simulink model "lab322"  (R2022a)
settings: Solver=VariableStepAuto  StartTime=0.0  StopTime=1  MaxStep=1e-3  RelTol=1e-3
undefined symbols (not defined in the file): ACsource, Angle, D1, lagging, Phase, pulse, RaLa, RbLb, RcLc, RL
libraries: spsThyristorLib x6, spsFourierLib x5, spsVoltageMeasurementLib x5, spsSeriesRLCBranchLib x4, spsACVoltageSourceLib x3, spsCurrentMeasurementLib x2, spsGroundLib x1, spsRMSLib x1, simulink x1, spsPLL3phLib x1, spsPulseGeneratorThyristor12PulseLib x1, spsThreePhaseVIMeasurementLib x1
settings Model: Creator=Viktor  LastModifiedBy=админ
settings ModelReferenceCC: EnableRefExpFcnMdlSchedulingChecks=off
settings RTWCC: Description=Generic Real-Time Target  GPUComputeCapability=5.0

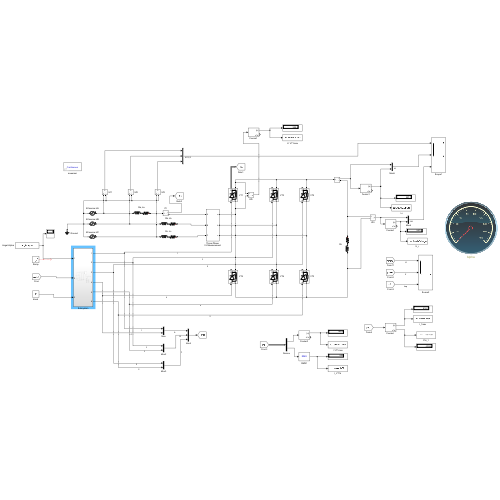
[thumbnail: Simulink's stored preview of the top-level diagram]
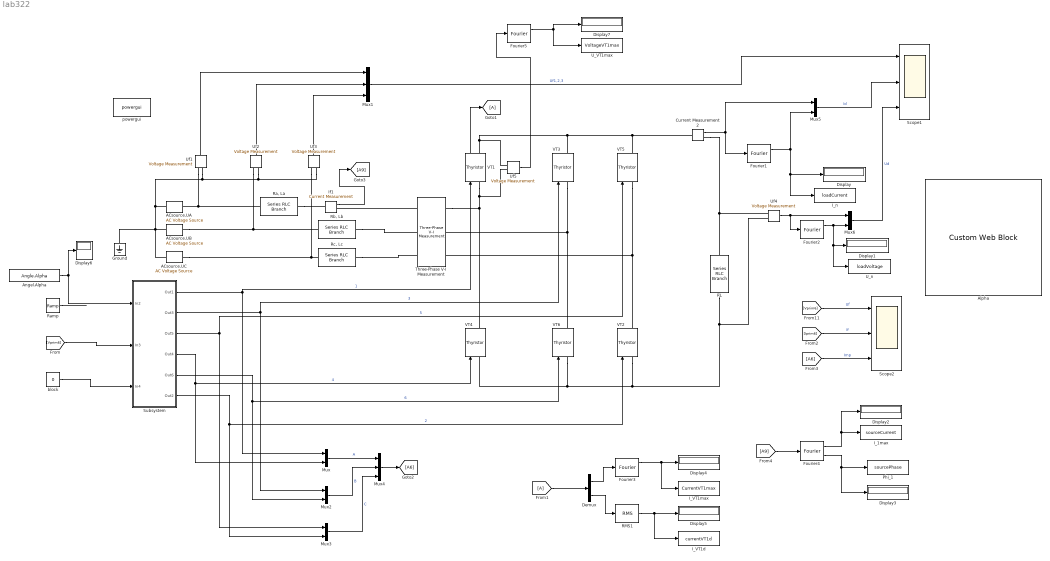
== system lab322 ==
  ACsource.UA : spsACVoltageSourceLib/AC Voltage Source  Amplitude=ACsource.U_A  Phase=Phase.A  Frequency=ACsource.f_c  SampleTime=0  Measurements=None  BusType=swing  Pref=10e3  Qref=0  Qmin=-inf  Qmax=+inf
  ACsource.UB : spsACVoltageSourceLib/AC Voltage Source  Amplitude=ACsource.U_B  Phase=Phase.B  Frequency=ACsource.f_c  SampleTime=0  Measurements=None  BusType=swing  Pref=10e3  Qref=0  Qmin=-inf  Qmax=+inf
  ACsource.UC : spsACVoltageSourceLib/AC Voltage Source  Amplitude=ACsource.U_C  Phase=Phase.C  Frequency=ACsource.f_c  SampleTime=0  Measurements=None  BusType=swing  Pref=10e3  Qref=0  Qmin=-inf  Qmax=+inf
  Alpha : CustomWebBlock  LabelPosition=Hide  ShowInitialText=on  Configuration="{\"components\":[{\"name\":\"CircularScaleComponent\",\"settings\":{\"bounds\":{\"max\":180,\"min\":0,\"tickInterval\":\"auto\"},\"direction\":\"cw\",\"flipLimits\":0,\"innerRadius\":0.75,\"internalTickHeightScaleFactor\":1,\"labelColor\":[255,255,200],\"labelFont\":{\"font\":\"Arial\",\"fontSize\":12},\"labelTransparency\":1,\"minorTickHeightScaleFactor\":0.2,\"needleImage\":{\"size\":[200,50],\"src\":\"data:image\\/svg+xml;base64,PD94bWwgdmVyc2lvbj0iMS4wIiBlbmNvZGluZz0idXRmLTgiPz4KPCEtLSBHZW5lcmF0b3I6IEFkb2JlIElsbHVzdHJhdG9yIDI0LjEuMiwgU1ZHIEV4cG9ydCBQbHVnLUluIC4gU1ZHIFZlcnNpb246IDYuMDAgQnVpbGQgMCkgIC0tPgo8c3ZnIHZlcnNpb249IjEuMSIgaWQ9IkxheWVyXzEiIHhtbG5zPSJodHRwOi8vd3d3LnczLm9yZy8yMDAwL3N2ZyIgeG1sbnM6eGxpbms9Imh0dHA6Ly93d3cudzMub3JnLzE5OTkveGxpbmsiIHg9IjBweCIgeT0iMHB4IgoJIHZpZXdCb3g9IjAgMCAyMDAgNTAiIHN0eWxlPSJlbmFibGUtYmFja2dyb3VuZDpuZXcgMCAwIDIwMCA1MDsiIHhtbDpzcGFjZT0icHJlc2VydmUiPgo8c3R5bGUgdHlwZT0idGV4dC9jc3MiPgoJLnN0MHtmaWxsOiNFQzIxMjc7fQo8L3N0eWxlPgo8cGF0aCBjbGFzcz0ic3QwIiBkPSJNMTYyLjgsMTMuN0MxNjksNC40LDE4MS43LDEuOSwxOTEsOC4xczExLjgsMTguOSw1LjYsMjguMnMtMTguOSwxMS44LTI4LjIsNS42bDAsMAoJQzE1OS4xLDM1LjYsMTU2LjYsMjMsMTYyLjgsMTMuN0wxNjIuOCwxMy43eiBNMTY1LjgsMTUuOGMtNS4xLDcuNi0zLjEsMTcuOSw0LjYsMjNjNy42LDUuMSwxNy45LDMuMSwyMy00LjYKCWM1LjEtNy42LDMuMS0xNy45LTQuNi0yM2wwLDBDMTgxLjIsNi4yLDE3MC45LDguMiwxNjUuOCwxNS44eiIvPgo8cGF0aCBjbGFzcz0ic3QwIiBkPSJNMC40LDI1Ljl2LTMuM2wxNTktMi41Yy0wLjcsMi42LTAuNyw1LjIsMCw3LjhMMC40LDI1Ljl6Ii8+CjxjaXJjbGUgY2xhc3M9InN0MCIgY3g9IjE3OS42IiBjeT0iMjQiIHI9IjAuNyIvPgo8L3N2Zz4K\"},\"needleOffset\":[0.18464878250906522,0],\"needleOrientation\":-45,\"needleRotation\":180,\"needleSize\":{\"height\":0.11741692305346914,\"width\":0.46108337545091255},\"outerRadius\":0.9,\"position\":[0.06486742424242424,0.05627705627705628,0.8917748917748918,0.8787878787878788],\"referencePoint\":\"auto\",\"scaleAngle\":270,\"scaleAngleOffset\":135,\"scaleColors\":[{\"color\":[162,20,47],\"max\":0,\"min\":0}],\"scaleColorsSize\":0.2,\"scaleDirection\":\"CW\",\"scalePosition\":[0,0,1,1],\"showLabels\":1,\"showMinorTicks\":1,\"showSpanLine\":1,\"showTicks\":1,\"tickColor\":[252,252,197],\"tickTransparency\":1,\"valueBarColor\":[217,83,25],\"valueBarPosition\":[0,0,1,1],\"valueBarSize\":0.2,\"valueBarTransparency\":1}},{\"name\":\"BackgroundImageComponent\",\"settings\":{\"image\":{\"size\":[500,500],\"src\":\"data:image\\/svg+xml;base64,PD94bWwgdmVyc2lvbj0iMS4wIiBlbmNvZGluZz0iVVRGLTgiIHN0YW5kYWxvbmU9Im5vIj8+CjxzdmcKICAgeG1sbnM6ZGM9Imh0dHA6Ly9wdXJsLm9yZy9kYy9lbGVtZW50cy8xLjEvIgogICB4bWxuczpjYz0iaHR0cDovL2NyZWF0aXZlY29tbW9ucy5vcmcvbnMjIgogICB4bWxuczpyZGY9Imh0dHA6Ly93d3cudzMub3JnLzE5OTkvMDIvMjItcmRmLXN5bnRheC1ucyMiCiAgIHhtbG5zOnN2Zz0iaHR0cDovL3d3dy53My5vcmcvMjAwMC9zdmciCiAgIHhtbG5zPSJodHRwOi8vd3d3LnczLm9yZy8yMDAwL3N2ZyIKICAgeG1sbnM6 ...(+9964 chars)\"},\"position\":[0,0,1,1],\"scaleMode\":\"0\"}},{\"name\":\"ForegroundImageComponent\",\"settings\":{\"image\":{\"size\":[0,0],\"src\":\"default\",\"srcOrientation\":[]},\"isForeground\":1,\"position\":[0,0,1,1],\"scaleMode\":\"0\"}}],\"settings\":{\"BindingType\":\"signal\",\"aspectRatio\":1.032258064516129,\"backgroundColor\":[0,0,0,\"1\"],\"backgroundOffset\":0.14,\"backgroundOpacity\":1,\"direction\":\"cw\",\"fixedAspectRatio\":\"on\",\"flipLimits\":0,\"orientation\":\"horizontal\",\"showBackgroundColor\":false,\"value\":0},\"type\":\"CircularGauge\"}"
  Angel.Alpha : Constant  Value=Angle.Alpha
  Current Measurement2 : spsCurrentMeasurementLib/Current Measurement  PhasorSimulation=off  OutputType=Complex  PSBequivalent=0
  Demux : Demux  Outputs=2
  Display{,1..7} (8 alike) : Display
  Fourier1 : spsFourierLib/Fourier  Freq=ACsource.f_c  n=0  InInit=[0, 0]  Ts=0
      settings: SourceProductBaseCode=PS
  Fourier2 : spsFourierLib/Fourier  Freq=ACsource.f_c  n=0  InInit=[0, 0]  Ts=0
      settings: SourceProductBaseCode=PS
  Fourier3 : spsFourierLib/Fourier  Freq=ACsource.f_c  n=0  InInit=[0, 0]  Ts=0
      settings: SourceProductBaseCode=PS
  Fourier4 : spsFourierLib/Fourier  Freq=ACsource.f_c  n=1  InInit=[0, 0]  Ts=0
      settings: SourceProductBaseCode=PS
  Fourier5 : spsFourierLib/Fourier  Freq=ACsource.f_c  n=1  InInit=[0, 0]  Ts=0
      settings: SourceProductBaseCode=PS
  From1 : From
  Goto1 : Goto
  Ground : spsGroundLib/Ground  LConnTagsString=a
  I_1max : ToWorkspace  VariableName=sourceCurrent  SampleTime=-1
  I_VT1d : ToWorkspace  VariableName=currentVT1d  SampleTime=-1
  I_VT1max : ToWorkspace  VariableName=CurrentVT1max  SampleTime=-1
  I_n : ToWorkspace  VariableName=loadCurrent  SampleTime=-1
  If1 : spsCurrentMeasurementLib/Current Measurement  PhasorSimulation=off  OutputType=Complex  PSBequivalent=0
  Mux{,2..3,5..6} (5 alike) : Mux  Inputs=2
  Mux1 : Mux  Inputs=3
  Mux4 : Mux  Inputs=3
  Phi_1 : ToWorkspace  VariableName=sourcePhase  SampleTime=-1
      settings: Save2DSignal=2-D array (concatenate along first dimension)
  RL : spsSeriesRLCBranchLib/Series RLC Branch  LConnTagsString=__new0  RConnTagsString=__new0  BranchType=RL  Resistance=RL.Res  Inductance=RL.Ind  SetiL0=off  InitialCurrent=0  Capacitance=1e-6  Setx0=off  InitialVoltage=0  Measurements=None
  RMS1 : spsRMSLib/RMS  TrueRMS=on  Freq=ACsource.U_A  RMSInit=0  Ts=0
  "Ra, La" : spsSeriesRLCBranchLib/Series RLC Branch  LConnTagsString=__new0  RConnTagsString=__new0  BranchType=RL  Resistance=RaLa.Res  Inductance=RaLa.Ind  SetiL0=off  InitialCurrent=0  Capacitance=1e-6  Setx0=off  InitialVoltage=0  Measurements=None
  Ramp : simulink/Sources/Ramp  slope=1  start=0  InitialOutput=0
  "Rb, Lb" : spsSeriesRLCBranchLib/Series RLC Branch  LConnTagsString=__new0  RConnTagsString=__new0  BranchType=RL  Resistance=RbLb.Res  Inductance=RbLb.Ind  SetiL0=off  InitialCurrent=0  Capacitance=1e-6  Setx0=off  InitialVoltage=0  Measurements=None
  "Rc, Lc" : spsSeriesRLCBranchLib/Series RLC Branch  LConnTagsString=__new0  RConnTagsString=__new0  BranchType=RL  Resistance=RcLc.Res  Inductance=RcLc.Ind  SetiL0=off  InitialCurrent=0  Capacitance=1e-6  Setx0=off  InitialVoltage=0  Measurements=None
  Scope1 : Scope  NumInputPorts=3
  Scope2 : Scope  NumInputPorts=3
  Subsystem : Subsystem
  Three-Phase V-I Measurement : spsThreePhaseVIMeasurementLib/Three-Phase V-I Measurement  VoltageMeasurement=phase-to-ground  SetLabelV=on  LabelV=Vprim6  Vpu=off  VpuLL=off  CurrentMeasurement=yes  SetLabelI=on  LabelI=Iprim6  Ipu=off  Pbase=100e6  Vbase=500e3  OutputType=Complex  PhasorSimulation=off  PSBequivalent=0
  U_VT1max : ToWorkspace  VariableName=VoltageVT1max  SampleTime=-1
  U_n : ToWorkspace  VariableName=loadVoltage  SampleTime=0.002
  Uf{1..5} (5 alike) : spsVoltageMeasurementLib/Voltage Measurement  PhasorSimulation=off  OutputType=Complex  PSBequivalent=0
  VT{1..6} (6 alike) : spsThyristorLib/Thyristor  Ron=VT.Res  Lon=0  Vf=VT.U_f  IC=0  Rs=500  Cs=250e-9  Measurements=on
  block : Constant  Value=0
  powergui : spspowerguiLib/powergui  Priority=1  SimulationMode=Continuous  SampleTime=50e-6  frequency=60  Iterations=50  frequencyindice=0  Pbase=100e6  ErrMax=1e-4  UnitsV=kV  UnitsW=MW  buscounter=0  FunctionMessages=off  echomessages=off  EnableUseOfTLC=off  CurrentSourceSwitches=off  DisableSnubberDevices=off  DisableRonSwitches=off  DisableVfSwitches=off  DisplayEquations=off  AutomaticDiscreteSolvers=off  SolverType=Tustin/Backward Euler (TBE)  Interpol=off  ExternalGateDelay=off  methode=off  Ts=100  x0status=blocks  SPID=on  SwTol=0  HookPort=off  NonlinearTolerance=1e-4  nMaxIteration=100  ContinueOnMaxIteration=off  RestoreLinks=warning  ResistiveCurrentMeasurement=off  Frange=[0:2:500]  Ylog=off  Xlog=on  ShowGrid=off  save=off  variable=ZData  structure=0  ZoomFFT=off  StartTime=0.0  cycles=1  DisplayStyle=1  fundamental=60  FreqAxis=off  MaxFrequency=1000  frequencyindicesteady=1  RmsSteady=1  display=off
  wires:
  Uf1/1 -> Mux1/1
  Uf2/1 -> Mux1/2
  Uf3/1 -> Mux1/3
  If1/1 -> [A9]
  Angel.Alpha/1 -> Subsystem/1(In2), Display6/1
  block/1 -> Subsystem/3(In4)
  [Vprim6] -> Subsystem/2(In3)
  Mux/1 -> Mux4/1  "A"
  Mux2/1 -> Mux4/2  "B"
  Mux3/1 -> Mux4/3  "C"
  Mux4/1 -> [A6]
  VT1/1 -> Goto1/1
  Current Measurement2/1 -> Fourier1/1, Mux5/1
  Fourier1/1 -> Mux5/2, Display/1, I_n/1
  Uf4/1 -> Fourier2/1, Mux6/1
  Fourier2/1 -> Display1/1, U_n/1, Mux6/2
  [Iprim6] -> Scope2/2  "If"
  [A6] -> Scope2/3  "Imp"
  [Vprim6] -> Scope2/1  "Uf"
  [A9] -> Fourier4/1
  Fourier4/1 -> I_1max/1, Display2/1
  Fourier4/2 -> Phi_1/1, Display3/1
  From1/1 -> Demux/1
  Demux/1 -> Fourier3/1
  Demux/2 -> RMS1/1
  Fourier3/1 -> I_VT1max/1, Display4/1
  RMS1/1 -> I_VT1d/1, Display5/1
  Ramp/1 -> ?
  Uf5/1 -> Fourier5/1
  Fourier5/1 -> U_VT1max/1, Display7/1
  Mux6/1 -> Scope1/3  "Ud"
  Mux5/1 -> Scope1/2  "Id"
  Mux1/1 -> Scope1/1  "Uf1,2,3"
  Subsystem/1(Out1) -> VT1/1, Mux/1  "1"
  Subsystem/2(Out3) -> VT3/1, Mux2/1  "3"
  Subsystem/3(Out5) -> VT5/1, Mux3/1  "5"
  Subsystem/6(Out2) -> Mux3/2, VT2/1  "2"
  Subsystem/5(Out6) -> Mux2/2, VT6/1  "6"
  Subsystem/4(Out4) -> Mux/2, VT4/1  "4"
  connections:
  "Ra, La"/RConn1 -- Uf1/LConn1 -- ACsource.UA/RConn1
  ACsource.UB/RConn1 -- Uf2/LConn1 -- "Rb, Lb"/RConn1
  ACsource.UC/RConn1 -- Uf3/LConn1 -- "Rc, Lc"/RConn1
  Ground/LConn1 -- ACsource.UC/LConn1 -- ACsource.UA/LConn1 -- Uf3/LConn2 -- Uf2/LConn2 -- Uf1/LConn2 -- ACsource.UB/LConn1
  "Ra, La"/LConn1 -- If1/LConn1
  Three-Phase V-I Measurement/LConn1 -- If1/RConn1
  VT1/LConn1 -- Uf5/LConn2 -- VT4/RConn1 -- Three-Phase V-I Measurement/RConn1
  VT3/LConn1 -- Three-Phase V-I Measurement/RConn2 -- VT6/RConn1
  VT5/LConn1 -- Three-Phase V-I Measurement/RConn3 -- VT2/RConn1
  VT1/RConn1 -- Uf5/LConn1 -- VT3/RConn1 -- VT5/RConn1 -- Current Measurement2/LConn1
  Current Measurement2/RConn1 -- Uf4/LConn1 -- RL/LConn1
  RL/RConn1 -- Uf4/LConn2 -- VT2/LConn1 -- VT6/LConn1 -- VT4/LConn1
  "Rb, Lb"/LConn1 -- Three-Phase V-I Measurement/LConn2
  "Rc, Lc"/LConn1 -- Three-Phase V-I Measurement/LConn3

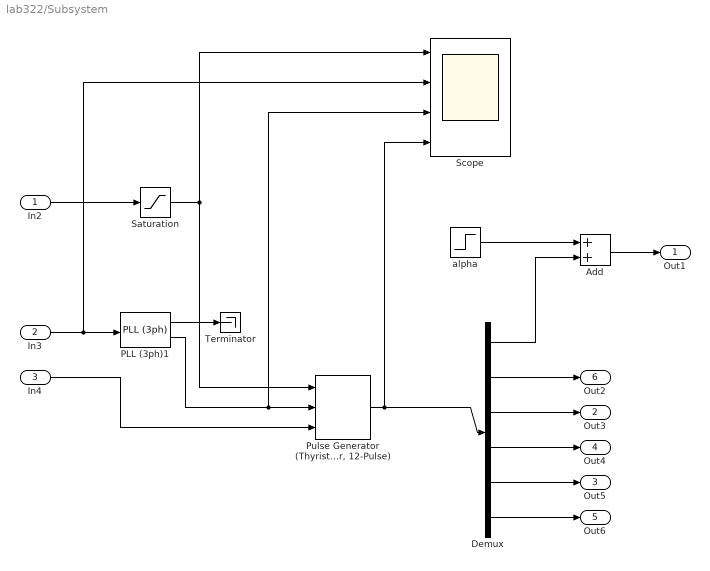
== system lab322/Subsystem ==
  In2 : Inport
  In3 : Inport  Port=2
  In4 : Inport  Port=3
  Add : Sum
  Demux : Demux  Outputs=6
  PLL (3ph)1 : spsPLL3phLib/PLL (3ph)  Fmin=45  Par_Init=[0, ACsource.f_c]  ParK=[180, 3200, 1]  TcD=1e-4  MaxRateChangeFreq=12  FilterCutOffFreq=25  Ts=0.0001  AGC=on
  "Pulse Generator (Thyristor, 12-Pulse)" : spsPulseGeneratorThyristor12PulseLib/Pulse Generator (Thyristor, 12-Pulse)  GenType=6-pulse  Delta=D1 (lagging)  pwidth=10  Double_Pulse=off  Ts=0.0001
      settings: SourceProductBaseCode=PS
  Saturation : Saturate  UpperLimit=120  LowerLimit=0
  Scope : Scope  NumInputPorts=4
  Terminator : Terminator
  alpha : Step  Time=1/ACsource.f_c/2  Before=1  After=0  SampleTime=0.0001
  Out1 : Outport
  Out3 : Outport  Port=2
  Out5 : Outport  Port=3
  Out4 : Outport  Port=4
  Out6 : Outport  Port=5
  Out2 : Outport  Port=6
  wires:
  In3/1 -> PLL (3ph)1/1, Scope/2
  PLL (3ph)1/2 -> "Pulse Generator (Thyristor, 12-Pulse)"/2, Scope/3
  In2/1 -> Saturation/1
  In4/1 -> "Pulse Generator (Thyristor, 12-Pulse)"/3
  Saturation/1 -> Scope/1, "Pulse Generator (Thyristor, 12-Pulse)"/1
  "Pulse Generator (Thyristor, 12-Pulse)"/1 -> Demux/1, Scope/4
  PLL (3ph)1/1 -> Terminator/1
  Demux/5 -> Out5/1
  Demux/6 -> Out6/1
  Demux/4 -> Out4/1
  Demux/3 -> Out3/1
  Demux/2 -> Out2/1
  alpha/1 -> Add/1
  Demux/1 -> Add/2
  Add/1 -> Out1/1
